simulink model "Problem_5"  (R2020a)
settings: Solver=VariableStepAuto  StartTime=0.0  StopTime=10.0  RelTol=1e-3
settings Model: Creator=Admin  LastModifiedBy=Admin

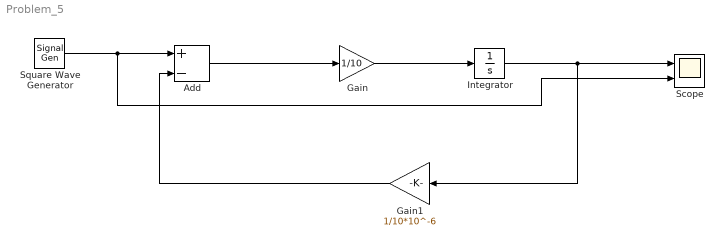
== system Problem_5 ==
  Add : Sum  Inputs=+-
  Gain : Gain  Gain=1/10
  Gain1 : Gain  Gain=1/10*10^-6
  Integrator : Integrator  InitialCondition=[0.000001 0.000002 0.000003 0.000004]
  Scope : Scope  NumInputPorts=2
  Square Wave Generator : SignalGenerator  WaveForm=square  Units=rad/sec
  wires:
  Add/1 -> Gain/1
  Gain1/1 -> Add/2
  Gain/1 -> Integrator/1
  Integrator/1 -> Scope/1, Gain1/1
  Square Wave Generator/1 -> Scope/2, Add/1
